simulink model "test_model"  (R2024b)
settings: Solver=VariableStepAuto  StartTime=6.69  StopTime=11.57  MaxStep=0.001  RelTol=1e-3  AbsTol=1e-3
values from neighbouring files (symbols this model uses):
  Fa = ec1807kf(ndx1,6)    [exp_data.m]
  Sd = ec1807kf(ndx1,2)    [exp_data.m]    (also in ga_optim.m = interp1(t, Sd, Tt1))
  tt = ec1807kf(ndx1,1)    [exp_data.m]
  Va = ec1807k(ndx1,6)    [exp_data.m]
  Xd = ec1807kf(ndx1,3)    [exp_data.m]    (also in ga_optim.m = interp1(t, Xd, Tt1))
settings Model: Creator=tsvetan  LastModifiedBy=tsvetan

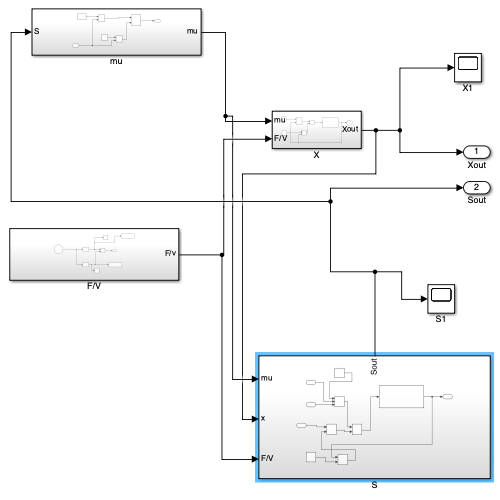
[thumbnail: Simulink's stored preview of the top-level diagram]
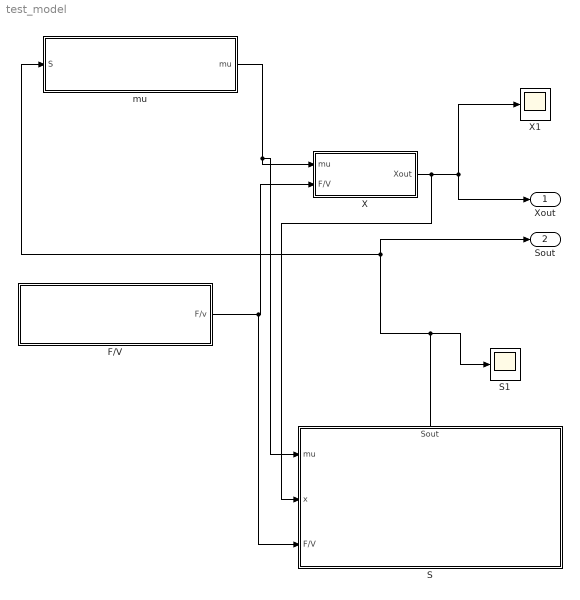
== system test_model ==
  F/V : Subsystem
  S : Subsystem
      settings: PortSchema="{\"entries\":[{\"content\":{\"sides\":[{\"content\":{\"connectorIds\":[\"In1\",\"In2\",\"In3\"]},\"type\":\"ConnectorPlacement.EquallySpacedRectSide\",\"uuid\":\"9a74bdac-b548-4137-a032-9cac2d72be40\"},{\"content\":{\"side\":\"RIGHT\"},\"type\":\"ConnectorPlacement.EquallySpacedRectSide\",\"uuid\":\"d4c5fdef-27ac-445a-8b9e-624041f2cb6b\"},{\"content\":{\"connectorIds\":[\"Out1\"],\"side\":\"TOP\"},\"type\":\"ConnectorPlacement.EquallySpacedRectSide\",\"uuid\":\"f64280b4-11dd-425a-a38d-e1082428f02b\"}]},\"type\":\"ConnectorPlacement.EquallySpacedConnector\",\"uuid\":\"7ed3c4de-b00d-49a5-a814-e4370b0d1174\"}],\"packageUris\":[\"http://schema.mathworks.com/mf0/Connector/R2020b\"],\"version\":\"1.0\"}"
  S1 : Scope
  X : Subsystem
  X1 : Scope
  mu : Subsystem
  Xout : Outport
  Sout : Outport  Port=2
  wires:
  mu/1(mu) -> S/1(mu), X/1(mu)
  F/V/1(F/v) -> S/3(F/V), X/2(F/V)
  X/1(Xout) -> S/2(x), Xout/1, X1/1
  S/1(Sout) -> S1/1, Sout/1, mu/1(S)

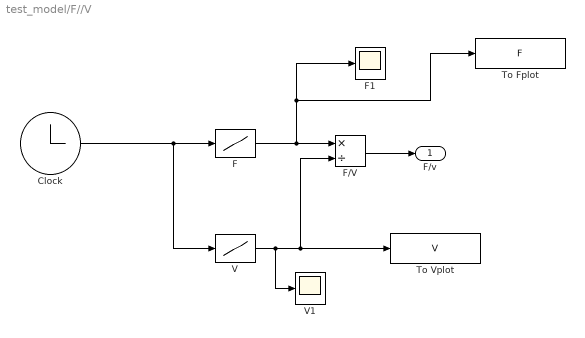
== system test_model/F//V ==
  Clock : Clock
  F : Lookup  InputValues=tt  Table=Fa
  F/V : Product  Inputs=*/
  F1 : Scope
  To Fplot : ToWorkspace  VariableName=F  SaveFormat=Timeseries  SampleTime=-1
  To Vplot : ToWorkspace  VariableName=V  SaveFormat=Timeseries  SampleTime=-1
  V : Lookup  InputValues=tt  Table=Va
  V1 : Scope
  F/v : Outport
  wires:
  Clock/1 -> F/1, V/1
  F/1 -> To Fplot/1, F1/1, F/V/1
  V/1 -> F/V/2, To Vplot/1, V1/1
  F/V/1 -> F/v/1

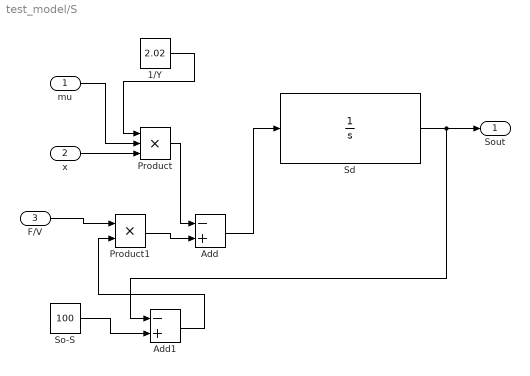
== system test_model/S ==
  mu : Inport
  x : Inport  Port=2
  F/V : Inport  Port=3
  1/Y : Constant  Value=2.02
  Add : Sum  Inputs=-+
  Add1 : Sum  Inputs=-+
  Product : Product  Inputs=3
  Product1 : Product
  Sd : Integrator  InitialCondition=Sd(1)
  So-S : Constant  Value=100
  Sout : Outport
  wires:
  x/1 -> Product/3
  mu/1 -> Product/2
  1/Y/1 -> Product/1
  Product/1 -> Add/1
  Product1/1 -> Add/2
  Add/1 -> Sd/1
  Sd/1 -> Add1/1, Sout/1
  F/V/1 -> Product1/1
  So-S/1 -> Add1/2
  Add1/1 -> Product1/2

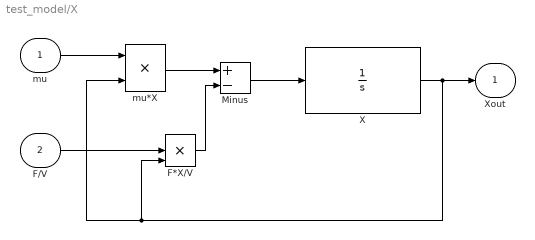
== system test_model/X ==
  mu : Inport
  F/V : Inport  Port=2
  F*X/V : Product  Inputs=3
  Minus : Sum  Inputs=+-
  X : Integrator  InitialCondition=Xd(1)
  mu*X : Product
  Xout : Outport
  wires:
  mu/1 -> mu*X/1
  F/V/1 -> F*X/V/2
  mu*X/1 -> Minus/1
  F*X/V/1 -> Minus/2
  Minus/1 -> X/1
  X/1 -> Xout/1, mu*X/2, F*X/V/3

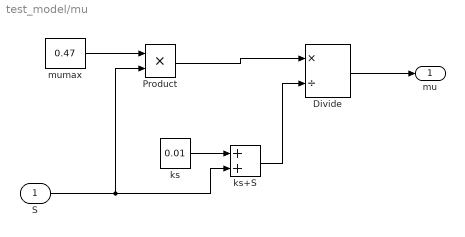
== system test_model/mu ==
  S : Inport
  Divide : Product  Inputs=*/
  Product : Product
  ks : Constant  Value=0.01
  ks+S : Sum
  mumax : Constant  Value=0.47
  mu : Outport
  wires:
  mumax/1 -> Product/1
  Product/1 -> Divide/1
  ks+S/1 -> Divide/2
  Divide/1 -> mu/1
  ks/1 -> ks+S/1
  S/1 -> ks+S/2, Product/2
